simulink library "mot"  (Simulink 8.1)
settings: Solver=ode1  StartTime=0.0  StopTime=Inf  FixedStep=0.001  RelTol=1e-3
PostLoadFcn:
  | , if any(exist('dsrtsu_mdlpostloadfcn', 'file') == [2, 3, 6]), try dsrtsu_mdlpostloadfcn('Execute', bdroot); catch fprintf('Error in PostLoadFcn (dsrtsu_mdlpostloadfcn) for model "%s":\n %s\n', bdroot, lasterr); end, end,
settings Model: DSRTSU_INTERNAL_RTI_VER=450  DSRTSU_INTERNAL_RTI_TYPE=rti1401  RTICANMMDATA=struct('GeneralSetupData',struct('modelroot','C:\Users\xsellart\Documents\TAIWAN_HAITEC\trunk\AdasDragon\software\sw_development\arch\app\per','generalsettings',struct('filesettings',struct('destfolder',struct('Name','RTICANMM_FILES','Check',1),'buildfolder',struct('Name','.','Check',1),'AbsDestfolder',struct('Name','C:\Users\xsellart\Documents\TAIWAN_HAITEC\trunk\AdasDragon\software\sw_development\arch\app\per\RTICANMM_FILES'),'AbsBuildfolder',struct('Name','C:\Users\xsellart\Documents\TAIWAN_HAITEC\trunk\AdasDragon\software\sw_development\arch\app\per'))),'options',struct('addpaths',1,'rmpaths',1,'addtrcexclusion',logical(1),'cannavigator',struct('checkmonitoring',0),'show_usrtrc',0,'use_usrtrc',0),'advanced',struct('options',[1 1 1 1 1 1 1 1 1 1 1 1 1 1 1 1 1 1 1 1 1 1 1 1 1 1 1 1 1 1 1 1 1 1 1 1 1 1 1 1 1 1 1 1 1 1 1 1 1 1 1 1 1 1 1 1 1 1 1 1 1 1 1 1 1 1 1 1 1 1 1 1 1 1 1 1 1 1 1 1 1 1 1 1 1 1 1 1 1 1 1 1 1 1 1 1 1 1 1 1]),'MPSetup',{{}},'modelname','mot','block','mot'))  DSRTSU_INTERNAL_RTIFPGA=40  Creator=xsellart  LastModifiedBy=xsellart

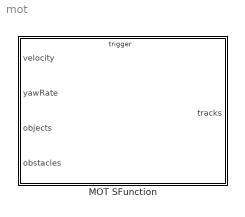
== system mot ==
  MOT SFunction : Subsystem  TreatAsAtomicUnit=on

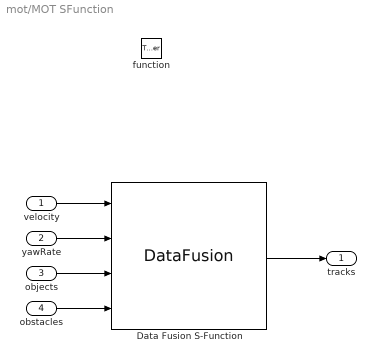
== system mot/MOT SFunction ==
  velocity : Inport
  yawRate : Inport  Port=2
  objects : Inport  Port=3
  obstacles : Inport  Port=4
  function : TriggerPort  TriggerType=function-call
  Data Fusion S-Function : S-Function  InitFcn=try, set_param(gcb,'FunctionName','DataFusion'), end  FunctionName=DataFusion  SFunctionModules=DataFusion_wrapper TrackingWrapper GeneratedCCode  WizardData=DataTag0  EnableBusSupport=off  mask(S-Function Builder){}
      mask help: Simulink:masks:SFunctionBuilder_MD
      mask init:
      | val = [[.9  0.75 0.75 1 1 .9 .9 1]',[1 1 0.75 0.75 .9 .9 1 .9]'];try , sys = get_param(gcb,'SfunBuilderFcnName');if isempty(sys), sys = get_param(gcb,'FunctionName'); end,catch, sys = get_param(gcb,'FunctionName'); end
      settings: CopyFcn=set_param(gcbh,'LinkStatus','none')  PreSaveFcn=try, set_param(gcb,'FunctionName','DataFusion'), end  OpenFcn=sfunctionwizard(gcbh)
      mask Display: plot(val(:,1),val(:,2)),disp(sys), port_label('input',1,'velocity'), port_label('input',2,'yawRate'), port_label('input',3,'objects'), port_label('input',4,'obstacles'), port_label('output',1,'tracks')
  tracks : Outport
  wires:
  velocity/1 -> Data Fusion S-Function/1
  obstacles/1 -> Data Fusion S-Function/4
  objects/1 -> Data Fusion S-Function/3
  yawRate/1 -> Data Fusion S-Function/2
  Data Fusion S-Function/1 -> tracks/1
